simulink model "circuit_analysis"  (R2020b)
settings: Solver=VariableStepAuto  StartTime=0.0  StopTime=10.0  RelTol=1e-3
settings Model: Creator=153  LastModifiedBy=153

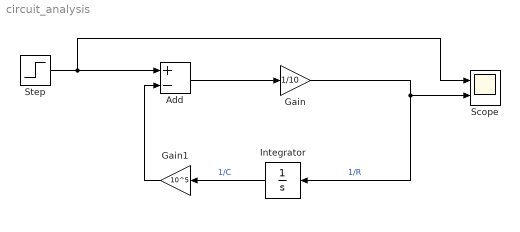
== system circuit_analysis ==
  Add : Sum  Inputs=+-
  Gain : Gain  Gain=1/10
  Gain1 : Gain  Gain=10^5
  Integrator : Integrator  InitialCondition=40
  Scope : Scope  NumInputPorts=2
  Step : Step  SampleTime=0
  wires:
  Add/1 -> Gain/1
  Gain/1 -> Scope/2, Integrator/1  "1/R"
  Step/1 -> Scope/1, Add/1
  Integrator/1 -> Gain1/1  "1/C"
  Gain1/1 -> Add/2
